simulink model "EncedidoLuces"  (R2022b)
settings: Solver=VariableStepAuto  StartTime=0.0  StopTime=inf  RelTol=1e-3
libraries: arduinolib x11, simulink x9
settings Model: Creator=laura  LastModifiedBy=laura

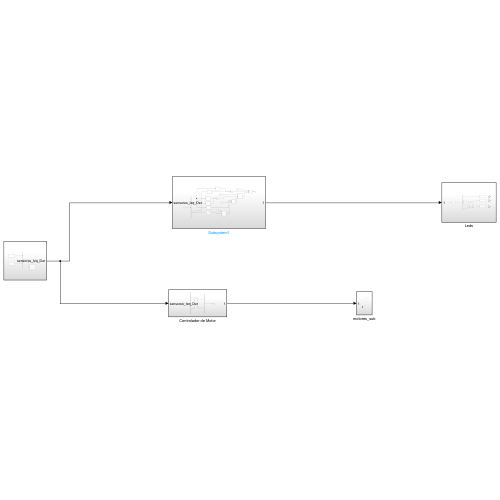
[thumbnail: Simulink's stored preview of the top-level diagram]
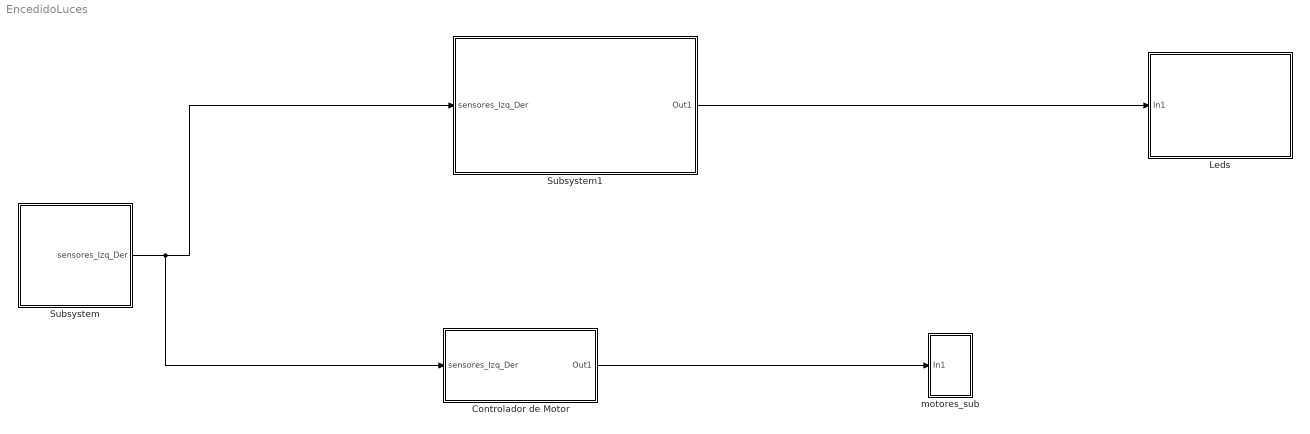
== system EncedidoLuces ==
  Controlador de Motor : Subsystem
  Leds : Subsystem
  Subsystem : Subsystem
  Subsystem1 : Subsystem
  motores_sub : Subsystem
  wires:
  Subsystem/1(sensores_Izq_Der) -> Controlador de Motor/1(sensores_Izq_Der), Subsystem1/1(sensores_Izq_Der)
  Subsystem1/1(Out1) -> Leds/1(In1)
  Controlador de Motor/1(Out1) -> motores_sub/1(In1)

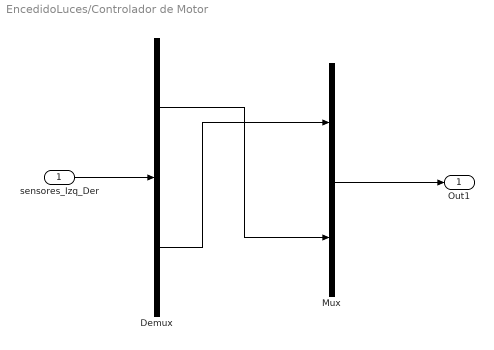
== system EncedidoLuces/Controlador de Motor ==
  sensores_Izq_Der : Inport
  Demux : Demux  Outputs=2
  Mux : Mux  Inputs=2
  Out1 : Outport
  wires:
  Demux/2 -> Mux/1
  Mux/1 -> Out1/1
  sensores_Izq_Der/1 -> Demux/1
  Demux/1 -> Mux/2

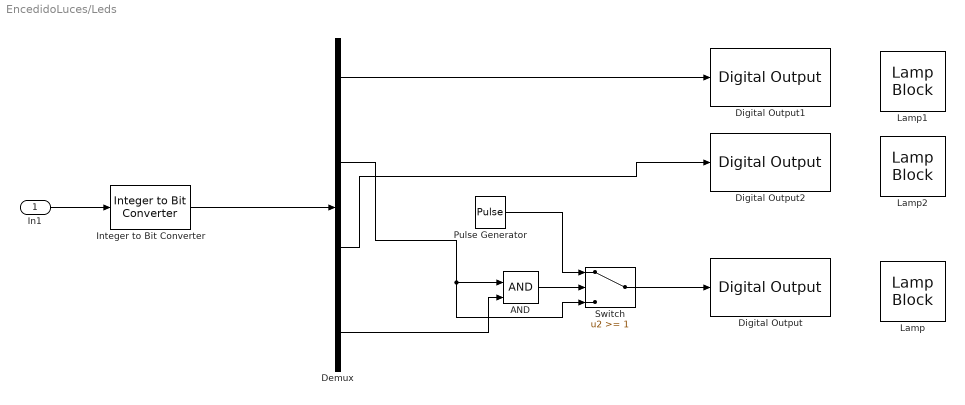
== system EncedidoLuces/Leds ==
  In1 : Inport
  AND : Logic  IconShape=distinctive  AllPortsSameDT=off  OutDataTypeStr=boolean
  Demux : Demux
  Digital Output : arduinolib/Digital Output  pinNumber=9  Direction=output  blockPlatform=arduino
  Digital Output1 : arduinolib/Digital Output  pinNumber=9  Direction=output  blockPlatform=arduino
  Digital Output2 : arduinolib/Digital Output  pinNumber=9  Direction=output  blockPlatform=arduino
  Integer to Bit Converter : simulink/Logic and Bit Operations/Integer to Bit Converter  nbits=4  signedInputValues=Unsigned  bitOrder=LSB first  outDtype=boolean
  Lamp : LampBlock  LabelPosition=Hide
  Lamp1 : LampBlock  LabelPosition=Hide
  Lamp2 : LampBlock  LabelPosition=Hide
  Pulse Generator : DiscretePulseGenerator  PulseType=Time based  Period=0.1  PulseWidth=50
  Switch : Switch  Threshold=1  SaturateOnIntegerOverflow=off  InputSameDT=off
  wires:
  Demux/4 -> AND/2
  AND/1 -> Switch/2
  Integer to Bit Converter/1 -> Demux/1
  Switch/1 -> Digital Output/1
  Pulse Generator/1 -> Switch/1
  Demux/2 -> Switch/3, AND/1
  Demux/1 -> Digital Output1/1
  Demux/3 -> Digital Output2/1
  In1/1 -> Integer to Bit Converter/1

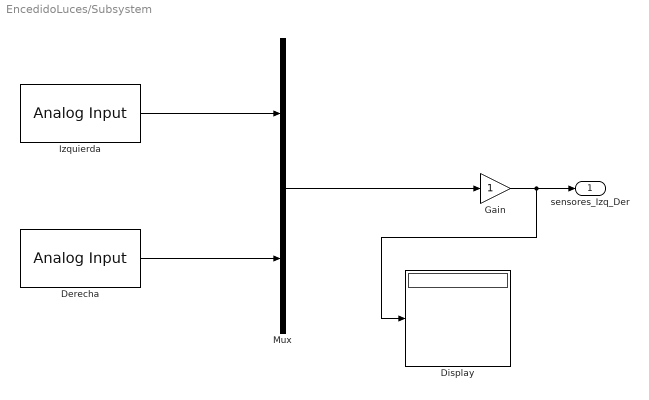
== system EncedidoLuces/Subsystem ==
  Derecha : arduinolib/Analog Input  pinNumber=1  ReadResultsOnly=off  ConversionTriggerSource=Software  ExternalTriggerType=uint32( 0 )  OutputDataType=uint16  EnableConversionCompleteNotify=off  EnableOuputStatus=off  SampleTime=0.1  blockPlatform=arduino
  Display : Display
  Gain : Gain
  Izquierda : arduinolib/Analog Input  pinNumber=0  ReadResultsOnly=off  ConversionTriggerSource=Software  ExternalTriggerType=uint32( 0 )  OutputDataType=uint16  EnableConversionCompleteNotify=off  EnableOuputStatus=off  SampleTime=0.1  blockPlatform=arduino
  Mux : Mux  Inputs=2
  sensores_Izq_Der : Outport
  wires:
  Mux/1 -> Gain/1
  Derecha/1 -> Mux/2
  Gain/1 -> Display/1, sensores_Izq_Der/1
  Izquierda/1 -> Mux/1

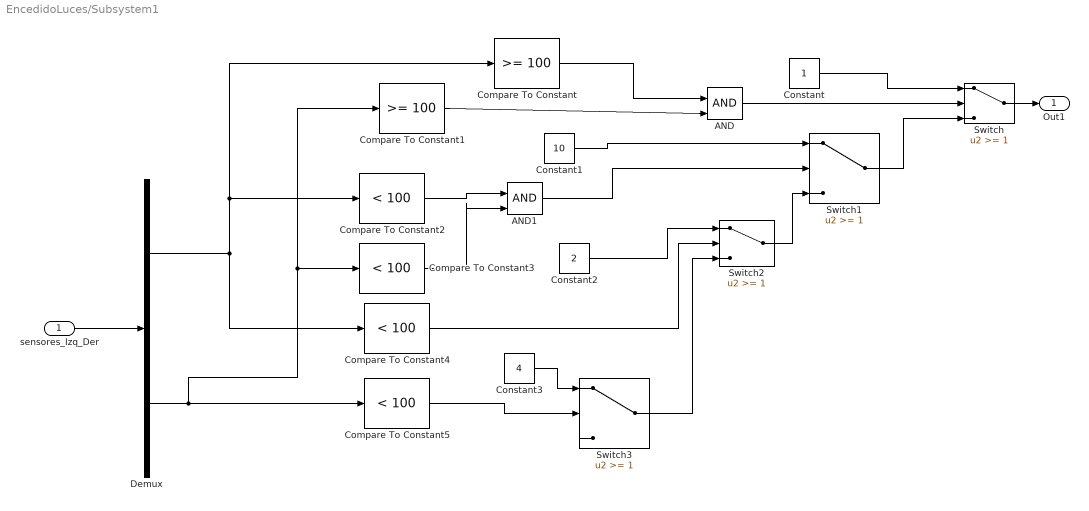
== system EncedidoLuces/Subsystem1 ==
  sensores_Izq_Der : Inport
  AND : Logic  IconShape=distinctive  AllPortsSameDT=off  OutDataTypeStr=boolean
  AND1 : Logic  IconShape=distinctive  AllPortsSameDT=off  OutDataTypeStr=boolean
  Compare To Constant : simulink/Logic and Bit Operations/Compare To Constant  relop=>=  const=100  OutDataTypeStr=boolean
  Compare To Constant1 : simulink/Logic and Bit Operations/Compare To Constant  relop=>=  const=100  OutDataTypeStr=boolean
  Compare To Constant{2..5} (4 alike) : simulink/Logic and Bit Operations/Compare To Constant  relop=<  const=100  OutDataTypeStr=boolean
  Constant : Constant
  Constant1 : Constant  Value=10
  Constant2 : Constant  Value=2
  Constant3 : Constant  Value=4
  Demux : Demux  Outputs=2
  Switch{,1..3} (4 alike) : Switch  Threshold=1  SaturateOnIntegerOverflow=off  InputSameDT=off
  Out1 : Outport
  wires:
  sensores_Izq_Der/1 -> Demux/1
  Demux/1 -> Compare To Constant/1, Compare To Constant2/1, Compare To Constant4/1
  Demux/2 -> Compare To Constant5/1, Compare To Constant3/1, Compare To Constant1/1
  Compare To Constant/1 -> AND/1
  Compare To Constant1/1 -> AND/2
  AND/1 -> Switch/2
  Constant/1 -> Switch/1
  Switch1/1 -> Switch/3
  Compare To Constant2/1 -> AND1/1
  Compare To Constant3/1 -> AND1/2
  AND1/1 -> Switch1/2
  Constant1/1 -> Switch1/1
  Compare To Constant4/1 -> Switch2/2
  Constant2/1 -> Switch2/1
  Switch2/1 -> Switch1/3
  Compare To Constant5/1 -> Switch3/2
  Constant3/1 -> Switch3/1
  Switch3/1 -> Switch2/3
  Switch/1 -> Out1/1

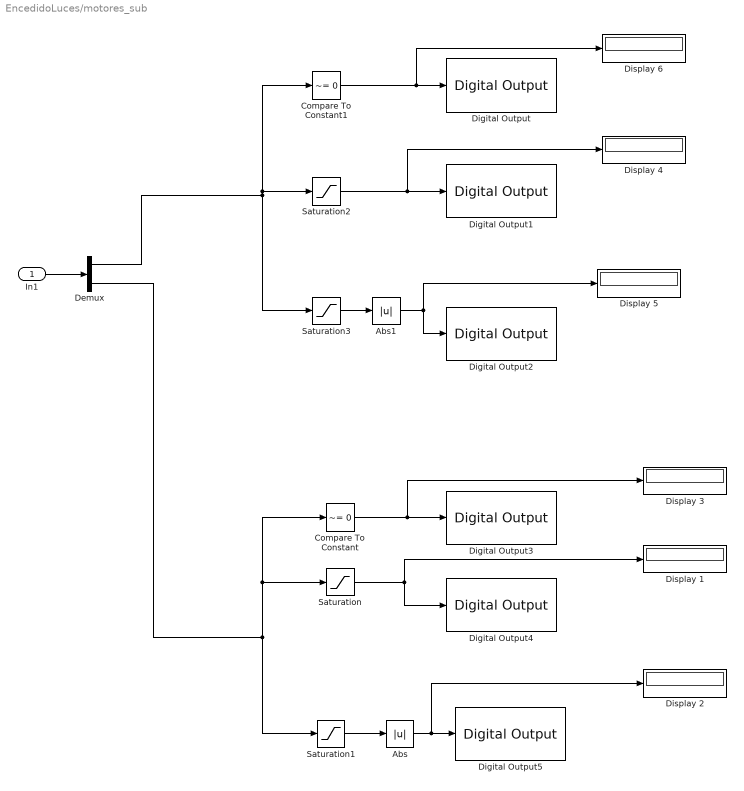
== system EncedidoLuces/motores_sub ==
  In1 : Inport
  Abs : Abs  SaturateOnIntegerOverflow=off
  Abs1 : Abs  SaturateOnIntegerOverflow=off
  Compare To Constant : simulink/Logic and Bit Operations/Compare To Constant  relop=~=  const=0  OutDataTypeStr=boolean
  Compare To Constant1 : simulink/Logic and Bit Operations/Compare To Constant  relop=~=  const=0  OutDataTypeStr=boolean
  Demux : Demux  Outputs=2
  Digital Output : arduinolib/Digital Output  pinNumber=9  Direction=output  blockPlatform=arduino
  Digital Output1 : arduinolib/Digital Output  pinNumber=11  Direction=output  blockPlatform=arduino
  Digital Output2 : arduinolib/Digital Output  pinNumber=13  Direction=output  blockPlatform=arduino
  Digital Output3 : arduinolib/Digital Output  pinNumber=15  Direction=output  blockPlatform=arduino
  Digital Output4 : arduinolib/Digital Output  pinNumber=17  Direction=output  blockPlatform=arduino
  Digital Output5 : arduinolib/Digital Output  pinNumber=19  Direction=output  blockPlatform=arduino
  Display {1..6} (6 alike) : Display
  Saturation{,1..3} (4 alike) : Saturate  UpperLimit=255  LowerLimit=1
  wires:
  Demux/1 -> Saturation3/1, Compare To Constant1/1, Saturation2/1
  Demux/2 -> Compare To Constant/1, Saturation/1, Saturation1/1
  Saturation1/1 -> Abs/1
  Compare To Constant/1 -> Digital Output3/1, Display 3/1
  Abs/1 -> Digital Output5/1, Display 2/1
  Abs1/1 -> Display 5/1, Digital Output2/1
  In1/1 -> Demux/1
  Saturation/1 -> Digital Output4/1, Display 1/1
  Saturation2/1 -> Display 4/1, Digital Output1/1
  Saturation3/1 -> Abs1/1
  Compare To Constant1/1 -> Digital Output/1, Display 6/1
